simulink model "messy_double_sensors"  (R2024b)
settings: Solver=VariableStepAuto  StartTime=0.0  StopTime=10.0  RelTol=1e-3
settings Model: Creator=giovanni  LastModifiedBy=giovanni
settings RTWCC: GPUComputeCapability=3.5

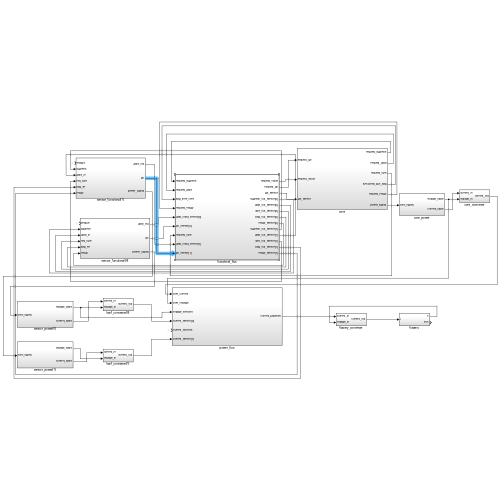
[thumbnail: Simulink's stored preview of the top-level diagram]
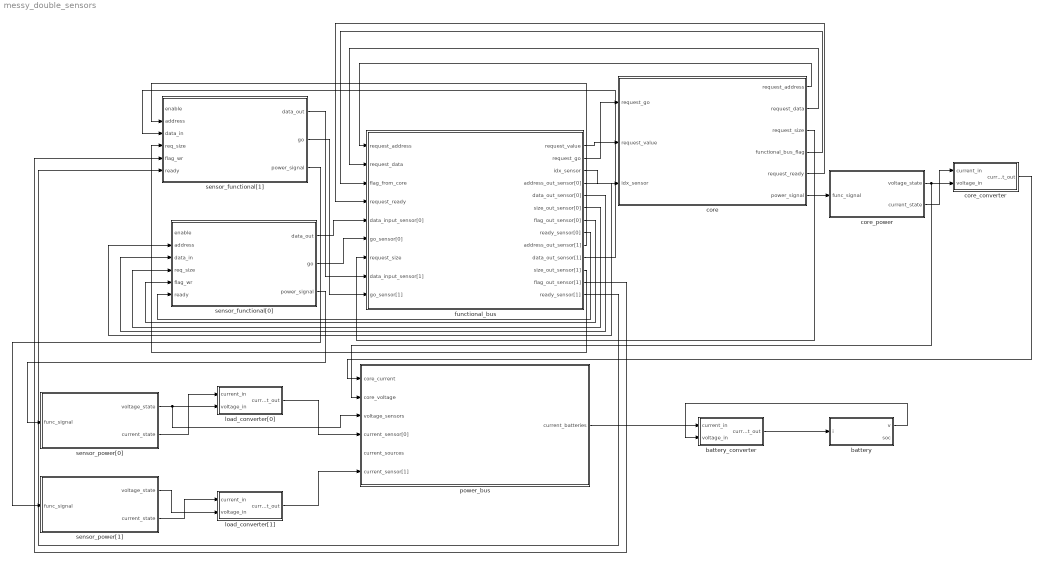
== system messy_double_sensors ==
  battery : Subsystem
  battery_converter : Subsystem
  core : Subsystem
  core_converter : Subsystem
  core_power : Subsystem
  functional_bus : Subsystem
  load_converter[0] : Subsystem
  load_converter[1] : Subsystem
  power_bus : Subsystem
  sensor_functional[0] : Subsystem
  sensor_functional[1] : Subsystem
  sensor_power[0] : Subsystem
  sensor_power[1] : Subsystem
  wires:
  battery/1(v) -> battery_converter/2(voltage_in)
  functional_bus/5(data_out_sensor[0]) -> sensor_functional[0]/3(data_in)
  functional_bus/6(size_out_sensor[0]) -> sensor_functional[0]/4(req_size)
  sensor_functional[0]/3(power_signal) -> sensor_power[0]/1(func_signal)
  power_bus/1(current_batteries) -> battery_converter/1(current_in)
  functional_bus/2(request_go) -> core/1(request_go)
  functional_bus/7(flag_out_sensor[0]) -> sensor_functional[0]/5(flag_wr)
  sensor_power[0]/2(current_state) -> load_converter[0]/1(current_in)
  load_converter[0]/1(current_out) -> power_bus/4(current_sensor[0])
  core_power/2(current_state) -> core_converter/1(current_in)
  core/6(power_signal) -> core_power/1(func_signal)
  sensor_power[0]/1(voltage_state) -> load_converter[0]/2(voltage_in), power_bus/3(voltage_sensors)
  core/3(request_size) -> functional_bus/7(request_size)
  functional_bus/1(request_value) -> core/2(request_value)
  functional_bus/8(ready_sensor[0]) -> sensor_functional[0]/6(ready)
  core/4(functional_bus_flag) -> functional_bus/3(flag_from_core)
  sensor_functional[0]/1(data_out) -> functional_bus/5(data_input_sensor[0])
  sensor_functional[0]/2(go) -> functional_bus/6(go_sensor[0])
  core_converter/1(current_out) -> power_bus/1(core_current)
  core_power/1(voltage_state) -> core_converter/2(voltage_in), power_bus/2(core_voltage)
  core/1(request_address) -> functional_bus/1(request_address)
  functional_bus/3(idx_sensor) -> core/3(idx_sensor)
  battery_converter/1(current_out) -> battery/1(i)
  core/5(request_ready) -> functional_bus/4(request_ready)
  core/2(request_data) -> functional_bus/2(request_data)
  functional_bus/4(address_out_sensor[0]) -> sensor_functional[0]/2(address)
  sensor_power[1]/2(current_state) -> load_converter[1]/1(current_in)
  sensor_power[1]/1(voltage_state) -> load_converter[1]/2(voltage_in)
  load_converter[1]/1(current_out) -> power_bus/6(current_sensor[1])
  sensor_functional[1]/3(power_signal) -> sensor_power[1]/1(func_signal)
  functional_bus/9(address_out_sensor[1]) -> sensor_functional[1]/2(address)
  functional_bus/10(data_out_sensor[1]) -> sensor_functional[1]/3(data_in)
  functional_bus/11(size_out_sensor[1]) -> sensor_functional[1]/4(req_size)
  functional_bus/12(flag_out_sensor[1]) -> sensor_functional[1]/5(flag_wr)
  functional_bus/13(ready_sensor[1]) -> sensor_functional[1]/6(ready)
  sensor_functional[1]/2(go) -> functional_bus/9(go_sensor[1])
  sensor_functional[1]/1(data_out) -> functional_bus/8(data_input_sensor[1])

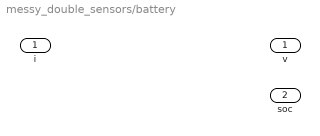
== system messy_double_sensors/battery ==
  i : Inport
  v : Outport
  soc : Outport  Port=2

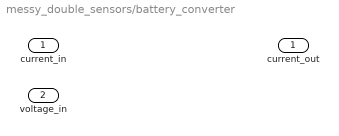
== system messy_double_sensors/battery_converter ==
  current_in : Inport
  voltage_in : Inport  Port=2
  current_out : Outport

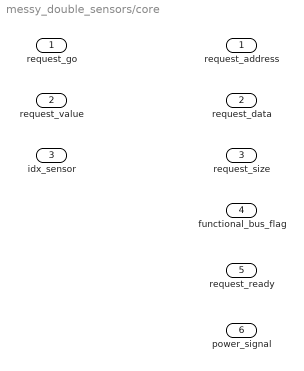
== system messy_double_sensors/core ==
  request_go : Inport
  request_value : Inport  Port=2
  idx_sensor : Inport  Port=3
  request_address : Outport
  request_data : Outport  Port=2
  request_size : Outport  Port=3
  functional_bus_flag : Outport  Port=4
  request_ready : Outport  Port=5
  power_signal : Outport  Port=6

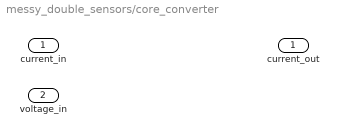
== system messy_double_sensors/core_converter ==
  current_in : Inport
  voltage_in : Inport  Port=2
  current_out : Outport

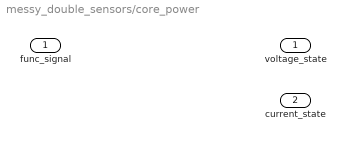
== system messy_double_sensors/core_power ==
  func_signal : Inport
  voltage_state : Outport
  current_state : Outport  Port=2

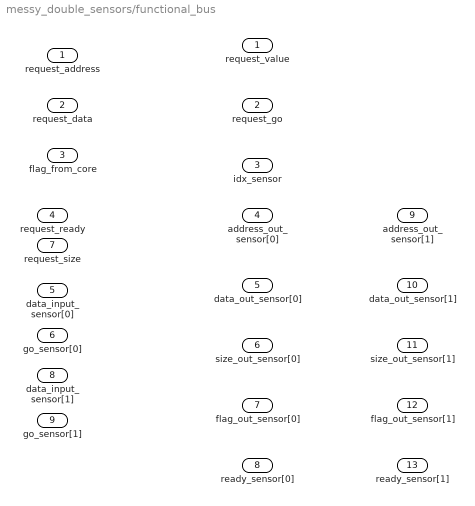
== system messy_double_sensors/functional_bus ==
  request_address : Inport
  request_data : Inport  Port=2
  flag_from_core : Inport  Port=3
  request_ready : Inport  Port=4
  data_input_sensor[0] : Inport  Port=5
  go_sensor[0] : Inport  Port=6
  request_size : Inport  Port=7
  data_input_sensor[1] : Inport  Port=8
  go_sensor[1] : Inport  Port=9
  request_value : Outport
  request_go : Outport  Port=2
  idx_sensor : Outport  Port=3
  address_out_sensor[0] : Outport  Port=4
  data_out_sensor[0] : Outport  Port=5
  size_out_sensor[0] : Outport  Port=6
  flag_out_sensor[0] : Outport  Port=7
  ready_sensor[0] : Outport  Port=8
  address_out_sensor[1] : Outport  Port=9
  data_out_sensor[1] : Outport  Port=10
  size_out_sensor[1] : Outport  Port=11
  flag_out_sensor[1] : Outport  Port=12
  ready_sensor[1] : Outport  Port=13

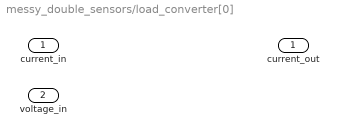
== system messy_double_sensors/load_converter[0] ==
  current_in : Inport
  voltage_in : Inport  Port=2
  current_out : Outport

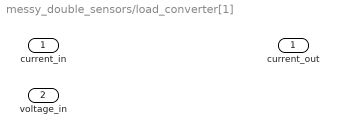
== system messy_double_sensors/load_converter[1] ==
  current_in : Inport
  voltage_in : Inport  Port=2
  current_out : Outport

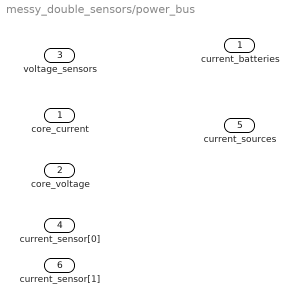
== system messy_double_sensors/power_bus ==
  core_current : Inport
  core_voltage : Inport  Port=2
  voltage_sensors : Inport  Port=3
  current_sensor[0] : Inport  Port=4
  current_sources : Inport  Port=5
  current_sensor[1] : Inport  Port=6
  current_batteries : Outport

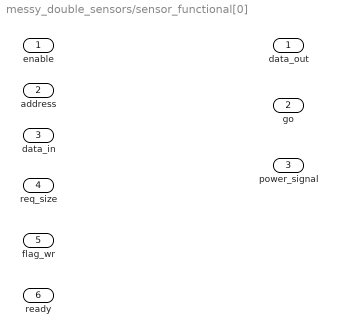
== system messy_double_sensors/sensor_functional[0] ==
  enable : Inport
  address : Inport  Port=2
  data_in : Inport  Port=3
  req_size : Inport  Port=4
  flag_wr : Inport  Port=5
  ready : Inport  Port=6
  data_out : Outport
  go : Outport  Port=2
  power_signal : Outport  Port=3

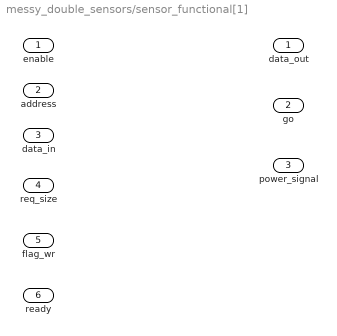
== system messy_double_sensors/sensor_functional[1] ==
  enable : Inport
  address : Inport  Port=2
  data_in : Inport  Port=3
  req_size : Inport  Port=4
  flag_wr : Inport  Port=5
  ready : Inport  Port=6
  data_out : Outport
  go : Outport  Port=2
  power_signal : Outport  Port=3

== system messy_double_sensors/sensor_power[0] ==
  func_signal : Inport
  voltage_state : Outport
  current_state : Outport  Port=2

== system messy_double_sensors/sensor_power[1] ==
  func_signal : Inport
  voltage_state : Outport
  current_state : Outport  Port=2
